simulink model "c3_lining_model"  (R2022a)
settings: Solver=VariableStepAuto  StartTime=0.0  StopTime=10.0  RelTol=1e-3
InitFcn:
  | uav_param
undefined symbols (not defined in the file or in its folder): gr_eff, uav_P
settings Model: Creator=Abhi  LastModifiedBy=Abhi

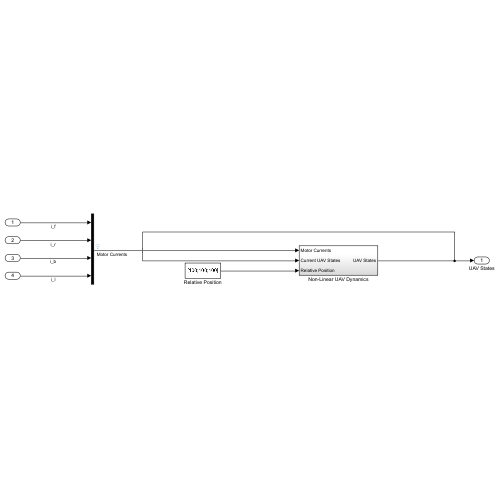
[thumbnail: Simulink's stored preview of the top-level diagram]
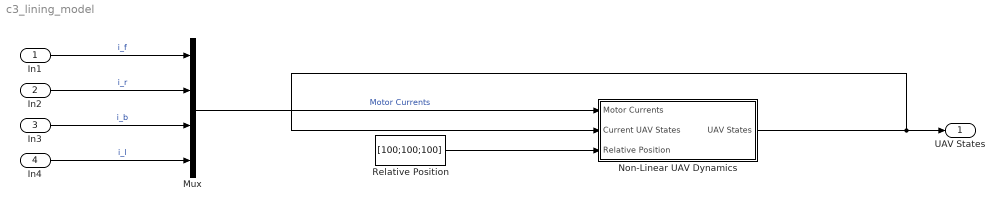
== system c3_lining_model ==
  In1 : Inport
  In2 : Inport  Port=2
  In3 : Inport  Port=3
  In4 : Inport  Port=4
  Mux : Mux
  Non-Linear UAV Dynamics : Subsystem
  Relative Position : Constant  Value=[100;100;100]
  UAV States : Outport
  wires:
  Relative Position/1 -> Non-Linear UAV Dynamics/3(Relative Position)
  Non-Linear UAV Dynamics/1(UAV States) -> Non-Linear UAV Dynamics/2(Current UAV States), UAV States/1
  In2/1 -> Mux/2  "i_r"
  In4/1 -> Mux/4  "i_l"
  In3/1 -> Mux/3  "i_b"
  In1/1 -> Mux/1  "i_f"
  Mux/1 -> Non-Linear UAV Dynamics/1(Motor Currents)  "Motor Currents"

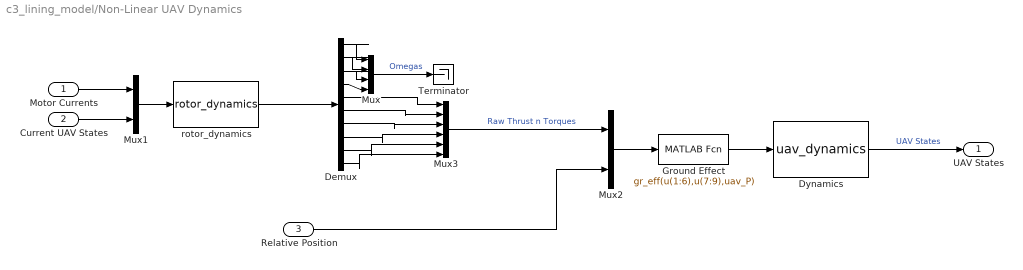
== system c3_lining_model/Non-Linear UAV Dynamics ==
  Motor Currents : Inport
  Current UAV States : Inport  Port=2
  Relative Position : Inport  Port=3
  Demux : Demux  Outputs=10
  Dynamics : S-Function  FunctionName=uav_dynamics  Parameters=uav_P  SFunctionDeploymentMode=off  EnableBusSupport=off
  Ground Effect : MATLABFcn  MATLABFcn=gr_eff(u(1:6),u(7:9),uav_P)
  Mux : Mux
  Mux1 : Mux  Inputs=2
  Mux2 : Mux  Inputs=2
  Mux3 : Mux  Inputs=6
  Terminator : Terminator
  rotor_dynamics : S-Function  FunctionName=rotor_dynamics  Parameters=uav_P  SFunctionDeploymentMode=off  EnableBusSupport=off
  UAV States : Outport
  wires:
  Mux1/1 -> rotor_dynamics/1
  rotor_dynamics/1 -> Demux/1
  Ground Effect/1 -> Dynamics/1
  Motor Currents/1 -> Mux1/1
  Relative Position/1 -> Mux2/2
  Current UAV States/1 -> Mux1/2
  Dynamics/1 -> UAV States/1  "UAV States"
  Mux2/1 -> Ground Effect/1
  Demux/1 -> Mux/1
  Demux/2 -> Mux/2
  Demux/3 -> Mux/3
  Demux/4 -> Mux/4
  Mux/1 -> Terminator/1  "Omegas"
  Demux/5 -> Mux3/1
  Demux/6 -> Mux3/2
  Demux/7 -> Mux3/3
  Demux/8 -> Mux3/4
  Demux/9 -> Mux3/5
  Demux/10 -> Mux3/6
  Mux3/1 -> Mux2/1  "Raw Thrust n Torques"
